simulink library "MCHP_Blockset"  (Simulink 7.5)
settings: Solver=ode45  SolverMode=SingleTasking  StartTime=0.0  StopTime=10.0  RelTol=1e-3
InitFcn:
  | disp('MCHP_Blockset_Library_InitFunction');
undefined symbols (not defined in the file): A0, A2, AD0, AVdd, B1, B5, B9, C10, C2, CMP2A, CMP3A, CMP4A, EXTREF1, EXTREF2, gcbh, MaxPer, MCHP_ACC_SAMx_Callback, MCHP_ADC_Callback, MCHP_ADC_HighSpeed_SAR_Callback, MCHP_ADC_HighSpeed_SAR_dsPIC_Callback, MCHP_ADC_SAME5x_Callback, MCHP_AFEC_SAM7x_Callback, MCHP_BUS_I2C_MASTER_callback, MCHP_BUS_SPI_callback, MCHP_C_function_Call_callback, MCHP_CN_Callback, MCHP_COMPARATOR1_callback, MCHP_CompilerOptimisation_Callback, MCHP_DACC_SAMx_Callback, MCHP_Digital_Input_Callback, MCHP_Digital_Output_Read_Callback, MCHP_Digital_Output_Write_Callback, MCHP_Fun, MCHP_HighSpeed_AnalogComparator_Callback, MCHP_IC_Callback, MCHP_IdleTask_Callback, MCHP_Interrupt_Callback, MCHP_Master_Callback, MCHP_MCPWM_Callback, MCHP_MCU_LOAD_Callback, MCHP_MCU_OVERLOAD_Callback, MCHP_MSI_Callback, MCHP_OC_HW_Callback, MCHP_OC_SW_Callback, MCHP_OP_AMP_Callback, MCHP_OrderInOut, MCHP_PDEC_Callback, MCHP_PGA_Callback, MCHP_PWM_Callback, MCHP_PWM_HighSpeed_Override_Callback, MCHP_PWM_HS_FEP_Callback, MCHP_PWM_SAM7x_Callback, MCHP_PWM_SAM7x_Override_Callback, MCHP_QDEC_SAMx_Callback, MCHP_QEI_Callback, MCHP_Scheduler_Options_Callback, MCHP_SECONDARY_CORE_Callback, MCHP_Tasks_State_Callback, MCHP_TCC_PWM_Callback, MCHP_TIMER_Config_Callback ... (+18)
libraries: MCHP_Blockset x2
(part 6 of 9)

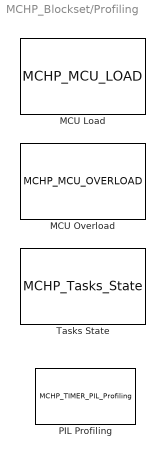
== system MCHP_Blockset/Profiling ==
  MCU Load : S-Function  InitFcn=MCHP_MCU_LOAD_Callback(gcbh,'InitFcn');  FunctionName=MCHP_MCU_LOAD  Parameters=[],MCHP_MCU_LOAD_Callback(gcbh,'S_OUTPUT'),[],MCHP_MCU_LOAD_Callback(gcbh,'S_OUTPUT_Size'),[],MCHP_MCU_LOAD_Callback(gcbh,'S_SampleTime'),0  EnableBusSupport=off  mask(MCU Load (Profile execution time)){MCULoadPin=Dynamic Options, MCULoadPin_TXT=A0 / Pin[17], MCULoadMeasure=on, TIMER_Resolution=Dynamic Options, TIMER_Resolution_TXT=Resol: 0.1143(us)  -  Max: 7.49(ms), MCHP_PORT={MCU Load Pin}{MCU_Load}0:1:A0;, MCHP_TIMER_REQUEST={MCU_Load}{MCU_Load}21:5:0:0:[]:524288;, MCHP_TIMER_RESULT=[2 65535 ], MCHP_MASTERLINK=UTester_33EP512MU810_CPULoad/Microchip Master, MCHP_COMPILED_INFO=CompiledSampleTime= [0.001   0 ];CompiledInportDataTypes=[ ];CompiledInportDataWidth=[];, Info=Timer 2:  Resol: 114.2857143(ns)  -  Max: 7.48983(ms), SampleTime=-1}
      mask prompts: MCULoadPin "MCU Load output PIN"; MCULoadMeasure "Output mcu load measurement"; TIMER_Resolution "Measure resolution"; Info "Timer info:"; SampleTime "Sample Time"
      mask help:
      | An output Pin is set high when CPU is busy: running time step calculation or a handling mcu interrupts.
      |
      | Busy time can be precisely quantified:
      | - in multitasking mode, the measurement trigger is the beginning of the task (sampling time) this block belong to.
      |
      | - in singletasking mode, the measurement trigger is the beginning of the groupe tasks which are triggered with this block.
      mask init:
      | MCHP_MCU_LOAD_Callback(gcbh,'INITIALISATION');
      settings: CopyFcn=MCHP_MCU_LOAD_Callback(gcbh,'CopyFcn');  PreSaveFcn=MCHP_Fun.PreSaveFcn_DynamicOptions(gcbh);  OpenFcn=MCHP_MCU_LOAD_Callback(gcbh,'OPEN');
      mask StyleString: popup(Dynamic Options),edit,checkbox,popup(Dynamic Options),edit,edit,edit,edit,edit,edit,edit,edit
      mask CallbackString: %MCHP_MCU_LOAD_Callback(gcbh,'MCULoadPin');||MCHP_MCU_LOAD_Callback(gcbh,'MCULoadMeasure');|MCHP_Fun.BlockUpdate(gcbh);||||||||
      mask Display:
      | MCHP_DrawLogo;disp('MCU Load\nLsb= 114.3(ns)\nA0');
      | port_label('output', 1 ,'L');
  MCU Overload : S-Function  InitFcn=MCHP_MCU_OVERLOAD_Callback(gcbh,'InitFcn');  FunctionName=MCHP_MCU_OVERLOAD  Parameters=[],MCHP_MCU_OVERLOAD_Callback(gcbh,'S_OUTPUT'),[],MCHP_MCU_OVERLOAD_Callback(gcbh,'S_OUTPUT_Size'),[],MCHP_MCU_OVERLOAD_Callback(gcbh,'S_SampleTime'),0  EnableBusSupport=off  mask(MCU Over-Load (Profile execution time)){MCUOverloadBlockOutput=on, MCUOverLoadPin=Dynamic Options, MCUOverLoadPin_TXT=None, MCHP_PORT=, MCHP_MASTERLINK=UTester_33EP512MU810_CPUOverLoad/Microchip Master, SampleTime=.001}
      mask prompts: MCUOverloadBlockOutput "Enable Block Output"; MCUOverLoadPin "MCU Overload PIN (asynchronously set to 1)"; SampleTime "Sample Time"
      mask help:
      | Block output is 0 when no overload has occured. Overload status is reset when block output is read.
      |
      | When an overload occurs, block output bit index represent overload for TID index.
      | bit 0 represent TID 0 (Fastest rate)
      | bit 1 represent TID 1 if it exist etc...
      | bit 15 represent TID 15 and higher
      |
      | Output pin is set to 1 asynchronously when an overload occurs. It remains equal to 1 and might be reset to 0 (Synchronously) using a digital Output block.
      mask init:
      | MCHP_MCU_OVERLOAD_Callback(gcbh,'INITIALISATION');
      settings: CopyFcn=MCHP_MCU_OVERLOAD_Callback(gcbh,'CopyFcn');  PreSaveFcn=MCHP_Fun.PreSaveFcn_DynamicOptions(gcbh);  OpenFcn=MCHP_MCU_OVERLOAD_Callback(gcbh,'OPEN');
      mask StyleString: checkbox,popup(Dynamic Options),edit,edit,edit,edit
      mask CallbackString: %MCHP_MCU_OVERLOAD_Callback(gcbh,'MCUOverloadBlockOutput');|%MCHP_MCU_OVERLOAD_Callback(gcbh,'MCUOverLoadPin');||||
      mask Display:
      | MCHP_DrawLogo;disp('MCU Over-Load');
      | port_label('output', 1 ,' ');
  PIL Profiling : S-Function  InitFcn=MCHP_TIMER_PIL_Profiling_Callback(gcbh,'InitFcn');  FunctionName=MCHP_TIMER_PIL_Profiling  EnableBusSupport=off  mask(Timer Configuration){TIMER_Ressource=Dynamic Options, TIMER_Ressource_TXT=No constraints [Prefered], TIMER_Ressource_Custom=[1], TIMER_Resolution=Dynamic Options, TIMER_Resolution_TXT=Resol: 32(us)  -  MaxPer: 2.1(s), MCHP_TIMER_REQUEST={TimerA}{TmrCfg}20:1:1:0:[]:4194304;, MCHP_TIMER_RESULT=[2 65535 ], MCHP_MASTERLINK=Timer_Config_30f4011/Microchip Master, Info=Timer 2}
      mask prompts: TIMER_Ressource "Timer Ressources"; TIMER_Ressource_TXT "Timer Ressources"; TIMER_Ressource_Custom "Timer List, example: [ 1  2  3  4  5 ]"; TIMER_Resolution "Resolution and max period"; Info "Timer info:"
      mask help:
      | Set Timer configuration
      | Peripheral that requrie a timer do not need this block. A timer is automatically assigned and configured in such case.
      mask init:
      | MCHP_TIMER_PIL_Profiling_Callback(gcbh,'INITIALISATION');
      settings: CopyFcn=MCHP_TIMER_PIL_Profiling_Callback(gcbh,'CopyFcn');  PreSaveFcn=MCHP_Fun.PreSaveFcn_DynamicOptions(gcbh);  OpenFcn=MCHP_TIMER_PIL_Profiling_Callback(gcbh,'OPEN');
      mask StyleString: popup(Dynamic Options),edit,edit,popup(Dynamic Options),edit,edit,edit,edit,edit
      mask CallbackString: MCHP_TIMER_PIL_Profiling_Callback(gcbh,'TIMER_Ressource');|||MCHP_TIMER_PIL_Profiling_Callback(gcbh,'TIMER_Resolution');|||||
      mask Display: MCHP_DrawLogo;disp('TIMER for PIL\nProfiling')
  Tasks State : S-Function  InitFcn=MCHP_Tasks_State_Callback(gcbh,'InitFcn');  FunctionName=MCHP_Tasks_State  Parameters=[],[],[],[],[],-1,0  EnableBusSupport=off  mask(MCU Over-Load (Profile execution time)){TasksPin=A[1:15], MCHP_PORT={Task D1 Running}{Task D1}15:1:A1;{Task D2 Running}{Task D2}15:1:A2;{Task D3 Running}{Task D3}15:1:A3;{Task D4 Running}{Task D4}15:1:A4;{Task D5 Running}{Task D5}15:1:A5;{Task D6 Running}{Task D6}15:1:A6;{Task D7 Running}{Task D7}15:1:A7;{Task D8 Running}{Task D8}15:1:A9;{Task D9 Running}{Task D9}15:1:A10;{Task D10 Running}{Task D10}15:1:A14;{Task D11 Running}{Task D11}15:1:A15;, MCHP_MASTERLINK=UTester_33EP512MU810_CPUOverLoad/Microchip Master}
      mask prompts: TasksPin "Running tasks pin list output ; example: A0 A1 A[5:8] B2..."
      mask help:
      | For each tasks, the corresponding pin is high when
      |  - the task is running or
      |  - the task execution is not finished but interrupted by an higher priority task
      | and set low otherwise
      |    First pin of the list is the state for the higher rate/priority task. (hit ctrl-j from model to show tasks list)
      | Value -1 will not affect a pin for the corresponding task.
      |
      | Task List updated with last model build
      | D1 => 1 (ms) ->  pin A1
      | D2 => 2 (ms) ->  pin A2
      | D3 => 4 (ms) ->  pin A3
      | D4 => 4  {+1} (ms) ->  pin A4
      | D5 => 20 (ms) ->  pin A5
      |
      | Available pins:
      |          A  [0   1   2   3   4   5   6   7   9  10  14  15]
      |          B  [0 : 15]
      |          C  [1   2   3   4  12  13  14  15]
      |          D  [0 : 15]
      |          E  [0 : 9]
      |          F  [0   1   2   3   4   5   8  12  13]
      |          G  [0   1   2   3   6   7   8   9  12  13  14  15]
      mask init:
      | MCHP_Tasks_State_Callback(gcbh,'INITIALISATION');
      settings: CopyFcn=MCHP_Tasks_State_Callback(gcbh,'CopyFcn');  OpenFcn=MCHP_Tasks_State_Callback(gcbh,'OPEN');
      mask Display: MCHP_DrawLogo;disp('Tasks State');

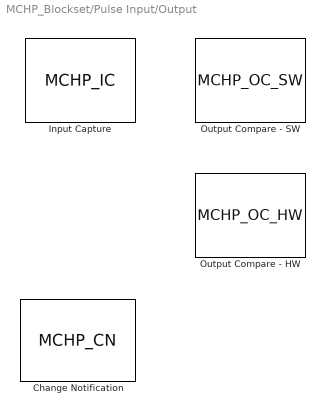
== system MCHP_Blockset/Pulse Input/Output ==
  Change Notification : S-Function  LoadFcn=MCHP_Fun.Load_EvalIn_ws(gcbh);  FunctionName=MCHP_CN  Parameters=SampleTime,MCHP_CN_Callback(gcbh,'S_INPUT'),MCHP_CN_Callback(gcbh,'S_OUTPUT'),0  EnableBusSupport=off  mask(Input driver for Change Notification Peripheral){IntPriority=6, Channel=[0     1     2], Channel_EP=[  C14  C13  B0 ], Channel_OLD=[0     1     2], Channel_UP_Down_Periode=[1     1     1], MaxChannel=[0.001   0.001   0.001], SafeMarge=[10    10    10], MaxChannelValue=2.^[ 13.966  13.966  13.966]  =>  [15999  15999  15999], CNxmax=[15999  15999  15999], Timer=[1  1  1], ChangeDetected=[0     0     0], OutputPortValue=[0     0     0], evalin_ws='', SampleTime=-1, Status=OK, MCHP_PORT={Change Notification 0}{CN0}9:0:C14;{Change Notification 1}{CN1}9:0:C13;{Change Notification 2}{CN2}9:0:B0;, MCHP_TIMER_REQUEST={Change Notification 0}{CN0}7:1:1:0:[]:17600;{Change Notification 1}{CN1}7:1:1:0:[]:17600;{Change Notification 2}{CN2}7:1:1:0:[]:17600;, MCHP_TIMER_RESULT=[2 17598.999999999996 ;2 17598.999999999996 ;2 17598.999999999996 ], MCHP_USER_INTERRUPTS={CNIE}{CN}{Change Notification}{6}, MCHP_MASTERLINK=Dvpt_CN/Microchip Master}
      mask prompts: IntPriority "Interrupt Priority  ( 1:lowest  7:Highest )"; Channel "CN Channels : [ 0  1  2  3  4  5  6  7 ]"; Channel_EP "CN Port : [  A0  A1  A2   ...   C7  C8  C9  ]"; Channel_OLD "internal"; Channel_UP_Down_Periode "Channel measurement type ; see above, within {1 2 3 4 5 8 10}"; MaxChannel "Max measured time / Channels"; SafeMarge "Safety margin in % (secure from overflow)"; MaxChannelValue "{'CN0max'  'CN1max'  'CN2max' } variables represent max time above ->"; CNxmax "CNxmax raw value"; ChangeDetected "Change Detected on   (0:None,  1:Rising edge, 2:Falling edge,  3:Both)"; OutputPortValue "Output Port Value"
      mask help:
      | Change Notification measure time :
      | 0 : no Measurements (for change detect only)
      | 1 : up
      | 2 : down
      | 3 : up & down
      | 4 : periode on rising edge
      | 8 : periode on falling edge
      | 5 : up & periode on rising edge
      | 10 : down & periode on falling edge
      |
      | CN Channels: [ 0  1  2  3  4  5  6  7 ]
      | CN Ports:      [  C14 C13 B0 B1 B2 B3 B4 B5 ]
      | CN Pins:       [ 16  15   2   3   4   5   6   7 ]
      mask init:
      | MCHP_CN_Callback(gcbh,'INITIALISATION');
      settings: PreSaveFcn=MCHP_Fun.PreSaveFcn_DynamicOptions(gcbh);  OpenFcn=MCHP_CN_Callback(gcbh,'OPEN');
      mask StyleString: popup(1|2|3|4|5|6|7),edit,edit,edit,edit,edit,edit,edit,edit,edit,edit,edit,edit,edit,edit,edit,edit,edit,edit,edit
      mask CallbackString: |MCHP_Fun.BlockUpdate(gcbh);|MCHP_Fun.BlockUpdate(gcbh);||MCHP_Fun.BlockUpdate(gcbh);||||||MCHP_Fun.BlockUpdate(gcbh);|MCHP_Fun.BlockUpdate(gcbh);||||||||
      mask Display:
      | MCHP_DrawLogo;color('blue');fprintf('CN        ');color('black');
      | 
      | port_label('output',1,'CN0_Up');
      | port_label('output',2,'CN1_Up');
      | port_label('output',3,'CN2_Up');
  Input Capture : S-Function  LoadFcn=MCHP_Fun.Load_EvalIn_ws(gcbh);  FunctionName=MCHP_IC  Parameters=SampleTime,MCHP_IC_Callback(gcbh,'S_INPUT'),MCHP_IC_Callback(gcbh,'S_OUTPUT'),0  EnableBusSupport=off  mask(Input driver for Input Capture Peripheral){IntPriority=4, Channel=[1     2], Channel_OLD=[1     2], PIN_IC1=Dynamic Options, PIN_IC1_TXT=Dynamic Options, PIN_IC2=Dynamic Options, PIN_IC2_TXT=Dynamic Options, PIN_IC3=Dynamic Options, PIN_IC3_TXT=Dynamic Options, PIN_IC4=Dynamic Options, PIN_IC4_TXT=Dynamic Options, PIN_IC5=Dynamic Options, PIN_IC5_TXT=Dynamic Options, PIN_IC6=Dynamic Options, PIN_IC6_TXT=Dynamic Options, PIN_IC7=Dynamic Options, PIN_IC7_TXT=Dynamic Options, PIN_IC8=Dynamic Options, PIN_IC8_TXT=Dynamic Options, PIN_IC9=Dynamic Options, PIN_IC9_TXT=Dynamic Options, PIN_IC10=Dynamic Options, PIN_IC10_TXT=Dynamic Options, PIN_IC11=Dynamic Options, PIN_IC11_TXT=Dynamic Options, PIN_IC12=Dynamic Options, PIN_IC12_TXT=Dynamic Options, PIN_IC13=Dynamic Options, PIN_IC13_TXT=Dynamic Options, PIN_IC14=Dynamic Options, PIN_IC14_TXT=Dynamic Options, PIN_IC15=Dynamic Options, PIN_IC15_TXT=Dynamic Options, PIN_IC16=Dynamic Options, PIN_IC16_TXT=Dynamic Options, Channel_UP_Down_Periode=[1     5], MaxChannel=[0.001     0.1], SafeMarge=[0     0], MaxChannelValue=2.^[ 7.960  14.610]  =>  [249  24999], ICxmax=[249  24999], Timer=[2  2], ChangeDetected=[0     0], ChangeDetectedPortRef=3, SampleTime=-1, evalin_ws='', Status=OK, MCHP_PORT={Input Capture 1}{IC1}6:0:D0;{Input Capture 2}{IC2}6:0:D1;, MCHP_TIMER_REQUEST={Input Capture 1}{IC1}6:1:1:0:[2  3]:16000;{Input Capture 2}{IC2}6:1:1:0:[2  3]:1600000;, MCHP_TIMER_RESULT=[2 15999 ;3 24999.000000000007 ], MCHP_MASTERLINK=Dvpt_IC/Microchip Master}
      mask prompts: IntPriority "Interrupt Priority  ( 1:lowest  7:Highest )"; Channel "Input Capture Channels : [ 1  2  7  8 ]"; Channel_OLD "internal"; PIN_IC1 "PIN for Input Capture 1 :"; PIN_IC1_TXT "internal"; PIN_IC2 "PIN for Input Capture 2 :"; PIN_IC2_TXT "internal"; PIN_IC3 "PIN for Input Capture 3 :"; PIN_IC3_TXT "internal"; PIN_IC4 "PIN for Input Capture 4 :"; PIN_IC4_TXT "internal"; PIN_IC5 "PIN for Input Capture 5 :"; PIN_IC5_TXT "internal"; PIN_IC6 "PIN for Input Capture 6 :"; PIN_IC6_TXT "internal"; PIN_IC7 "PIN for Input Capture 7 :"; PIN_IC7_TXT "internal"; PIN_IC8 "PIN for Input Capture 8 :"; PIN_IC8_TXT "internal"; PIN_IC9 "PIN for Input Capture 9 :"; PIN_IC9_TXT "internal"; PIN_IC10 "PIN for Input Capture 10 :"; PIN_IC10_TXT "internal"; PIN_IC11 "PIN for Input Capture 11 :"; PIN_IC11_TXT "internal"; PIN_IC12 "PIN for Input Capture 12 :"; PIN_IC12_TXT "internal"; PIN_IC13 "PIN for Input Capture 13 :"; PIN_IC13_TXT "internal"; PIN_IC14 "PIN for Input Capture 14 :"; PIN_IC14_TXT "internal"; PIN_IC15 "PIN for Input Capture 15 :"; PIN_IC15_TXT "internal"; PIN_IC16 "PIN for Input Capture 16 :"; PIN_IC16_TXT "internal"; Channel_UP_Down_Periode "Channel measurement type ; see above, within {1 2 3 4 5 8 10}"; MaxChannel "Max measured time / Channels"; SafeMarge "Safety margin in % (secure from overflow)"; MaxChannelValue "{'IC1max'  'IC2max' } variables represent max time above ->"; ICxmax "ICxmax raw value"; ChangeDetected "Change Detected on   (0:None,  1:Rising edge, 2:Falling edge,  3:Both)"
      mask help:
      | Input Capture measure time :
      | 0 : no Measurements (for change detect only)
      | 1 : up
      | 2 : down
      | 3 : up & down
      | 4 : periode on rising edge
      | 8 : periode on falling edge
      | 5 : up & periode on rising edge
      | 10 : down & periode on falling edge
      |
      | Input Capture Channels: [ 1  2  7  8 ]
      | Input Capture Ports:      [  D0 D1 B4 B5 ]
      | Input Capture Pins:       [ 23  18   6   7 ]
      mask init:
      | MCHP_IC_Callback(gcbh,'INITIALISATION');
      settings: PreSaveFcn=MCHP_Fun.PreSaveFcn_DynamicOptions(gcbh);  OpenFcn=MCHP_IC_Callback(gcbh,'OPEN');
      mask StyleString: popup(1|2|3|4|5|6|7),edit,edit,popup(Dynamic Options),edit,popup(Dynamic Options),edit,popup(Dynamic Options),edit,popup(Dynamic Options),edit,popup(Dynamic Options),edit,popup(Dynamic Options),edit,popup(Dynamic Options),edit,popup(Dynamic Options),edit,popup(Dynamic Options),edit,popup(Dynamic Options),edit,popup(Dynamic Options),edit,popup(Dynamic Options),edit,popup(Dynamic Options),edit,popup(Dynamic Options),edit,popup(Dynamic Options),edit,popup(Dynamic Options),edit,edit,edit,edit,edit,edit,edit,edit,edit,edit,edit,edit,edit,edit,edit,edit
      mask CallbackString:
      | |MCHP_Fun.BlockUpdate(gcbh);||if ~strcmp(get_param(gcbh,'PIN_IC1'),get_param(gcbh,'PIN_IC1_TXT'))
      | MCHP_Fun.BlockUpdate(gcbh);;
      | end||if ~strcmp(get_param(gcbh,'PIN_IC2'),get_param(gcbh,'PIN_IC2_TXT'))
      | MCHP_Fun.BlockUpdate(gcbh);;
      | end||if ~strcmp(get_param(gcbh,'PIN_IC3'),get_param(gcbh,'PIN_IC3_TXT'))
      | MCHP_Fun.BlockUpdate(gcbh);;
      | end||if ~strcmp(get_param(gcbh,'PIN_IC4'),get_param(gcbh,'PIN_IC4_TXT'))
      | MCHP_Fun.BlockUpdate(gcbh);;
      | end||if ~strcmp(get_param(gcbh,'PIN_IC5'),get_param(gcbh,'PIN_IC5_TXT'))
      | MCHP_Fun.BlockUpdate(gcbh);;
      | end||if ~strcmp(get_param(gcbh,'PIN_IC6'),get_param(gcbh,'PIN_IC6_TXT'))
      | MCHP_Fun.BlockUpdate(gcbh);;
      | end||if ~strcmp(get_param(gcbh,'PIN_IC7'),get_param(gcbh,'PIN_IC7_TXT'))
      | MCHP_Fun.BlockUpdate(gcbh);;
      | end||if ~strcmp(get_param(gcbh,'PIN_IC8'),get_param(gcbh,'PIN_IC8_TXT'))
      | MCHP_Fun.BlockUpdate(gcbh);;
      | end||if ~strcmp(get_param(gcbh,'PIN_IC9'),get_param(gcbh,'PIN_IC9_TXT'))
      | MCHP_Fun.BlockUpdate(gcbh);;
      | end||if ~strcmp(get_param(gcbh,'PIN_IC10'),get_param(gcbh,'PIN_IC10_TXT'))
      | MCHP_Fun.BlockUpdate(gcbh);;
      | end||if ~strcmp(get_param(gcbh,'PIN_IC11'),get_param(gcbh,'PIN_IC11_TXT'))
      | MCHP_Fun.BlockUpdate(gcbh);;
      | end||if ~strcmp(get_param(gcbh,'PIN_IC12'),get_param(gcbh,'PIN_IC12_TXT'))
      | MCHP_Fun.BlockUpdate(gcbh);;
      | end||if ~strcmp(get_param(gcbh,'PIN_IC13'),get_param(gcbh,'PIN_IC13_TXT'))
      | MCHP_Fun.BlockUpdate(gcbh);;
      | end||if ~strcmp(get_param(gcbh,'PIN_IC14'),get_param(gcbh,'PIN_IC14_TXT'))
      | MCHP_Fun.BlockUpdate(gcbh);;
      | end||if ~strcmp(get_param(gcbh,'PIN_IC15'),get_param(gcbh,'PIN_IC15_TXT'))
      | MCHP_Fun.BlockUpdate(gcbh);;
      | end||if ~strcmp(get_param(gcbh,'PIN_IC16'),get_param(gcbh,'PIN_IC16_TXT'))
      | MCHP_Fun.BlockUpdate(gcbh);;
      | end||MCHP_Fun.BlockUpdate(gcbh);||||||MCHP_Fun.BlockUpdate(gcbh);||||||||
      mask Display:
      | MCHP_DrawLogo;color('blue');fprintf('IC        ');color('black');
      | 
      | port_label('output',1,'IC1_Up');
      | port_label('output',2,'IC2_Up');
      | port_label('output',3,'IC2_Per');
  Output Compare - HW : S-Function  LoadFcn=MCHP_Fun.Load_EvalIn_ws(gcbh);  FunctionName=MCHP_OC_HW  Parameters=SampleTime,MCHP_OC_HW_Callback(gcbh,'S_INPUT'),MCHP_OC_HW_Callback(gcbh,'S_OUTPUT'),0  EnableBusSupport=off  mask(Input driver for Output Compare Peripheral Hardware){Channel=[1     2     3], Channel_OLD=[1     2     3], PIN_OC1_TXT=Dynamic Options, PIN_OC2_TXT=Dynamic Options, PIN_OC3_TXT=Dynamic Options, PIN_OC4_TXT=Dynamic Options, PIN_OC5_TXT=Dynamic Options, PIN_OC6_TXT=Dynamic Options, PIN_OC7_TXT=Dynamic Options, PIN_OC8_TXT=Dynamic Options, PIN_OC9_TXT=Dynamic Options, PIN_OC10_TXT=Dynamic Options, PIN_OC11_TXT=Dynamic Options, PIN_OC12_TXT=Dynamic Options, PIN_OC13_TXT=Dynamic Options, PIN_OC14_TXT=Dynamic Options, PIN_OC15_TXT=Dynamic Options, PIN_OC16_TXT=Dynamic Options, PIN_OCFA_TXT=Dynamic Options, PIN_OCFB_TXT=Dynamic Options, PIN_OCFC_TXT=Dynamic Options, Channel_UP_Down_Periode=[5    10     5], PulseTrig=Continuous pulses, InputPeriod=are set to the Max time (constant below), MaxChannel=[0.0001   0.0001   0.0001], MaxChannelUnique=.0001, MaxChannelValue=2.^[ 10.965  10.965  10.965]  =>  [1999  1999  1999], OCxmax=[1999  1999  1999], Timer=[-2 -2 -2], evalin_ws='', SampleTime=-1, MCHP_PORT={Output Compare 1}{OC1}7:1:P55;{Output Compare 2}{OC2}7:1:P56;{Output Compare 3}{OC3}7:1:P57;, MCHP_TIMER_REQUEST=, MCHP_TIMER_RESULT=[ ], MCHP_MASTERLINK=Dvpt_OC_HW/Microchip Master, PIN_OC1=Dynamic Options, PIN_OC2=Dynamic Options, PIN_OC3=Dynamic Options, PIN_OC4=Dynamic Options, PIN_OC5=Dynamic Options, PIN_OC6=Dynamic Options, PIN_OC7=Dynamic Options, PIN_OC8=Dynamic Options, PIN_OC9=Dynamic Options, PIN_OC10=Dynamic Options, PIN_OC11=Dynamic Options, PIN_OC12=Dynamic Options, PIN_OC13=Dynamic Options, PIN_OC14=Dynamic Options, PIN_OC15=Dynamic Options, PIN_OC16=Dynamic Options, PIN_OCFA=Dynamic Options, PIN_OCFB=Dynamic Options, PIN_OCFC=Dynamic Options}
      mask prompts: Channel "Output Compare Channels : [ 1  2  3  4 ]"; Channel_OLD "internal"; PIN_OC1_TXT "internal"; PIN_OC2_TXT "internal"; PIN_OC3_TXT "internal"; PIN_OC4_TXT "internal"; PIN_OC5_TXT "internal"; PIN_OC6_TXT "internal"; PIN_OC7_TXT "internal"; PIN_OC8_TXT "internal"; PIN_OC9_TXT "internal"; PIN_OC10_TXT "internal"; PIN_OC11_TXT "internal"; PIN_OC12_TXT "internal"; PIN_OC13_TXT "internal"; PIN_OC14_TXT "internal"; PIN_OC15_TXT "internal"; PIN_OC16_TXT "internal"; PIN_OCFA_TXT "internal"; PIN_OCFB_TXT "internal"; PIN_OCFC_TXT "internal"; Channel_UP_Down_Periode "Channel measurement type ; see above, within {5}"; PulseTrig "Mode"; InputPeriod "Period"; MaxChannel "Max time / Channels"; MaxChannelUnique "Max Time for all channels"; MaxChannelValue "{'OC1max'  'OC2max'  'OC3max' } variables represent max time above ->"; OCxmax "OCxmax raw value"; PIN_OC1 "PIN for Output Compare 1 :"; PIN_OC2 "PIN for Output Compare 2 :"; PIN_OC3 "PIN for Output Compare 3 :"; PIN_OC4 "PIN for Output Compare 4 :"; PIN_OC5 "PIN for Output Compare 5 :"; PIN_OC6 "PIN for Output Compare 6 :"; PIN_OC7 "PIN for Output Compare 7 :"; PIN_OC8 "PIN for Output Compare 8 :"; PIN_OC9 "PIN for Output Compare 9 :"; PIN_OC10 "PIN for Output Compare 10 :"; PIN_OC11 "PIN for Output Compare 11 :"; PIN_OC12 "PIN for Output Compare 12 :"; PIN_OC13 "PIN for Output Compare 13 :"; PIN_OC14 "PIN for Output Compare 14 :"; PIN_OC15 "PIN for Output Compare 15 :"; PIN_OC16 "PIN for Output Compare 16 :"; PIN_OCFA "PIN for Output Compare Fault A:"; PIN_OCFB "PIN for Output Compare Fault B:"; PIN_OCFC "PIN for Output Compare Fault C:"
      mask help:
      | Output Compare Setting :
      | 5 : up & periode
      | 10 : down & periode
      |
      |
      | Output Compare Channels: [ 1 2 3 4 ]
      | Output Compare Pins are remapables.
      mask init:
      | MCHP_OC_HW_Callback(gcbh,'INITIALISATION');
      settings: PreSaveFcn=MCHP_Fun.PreSaveFcn_DynamicOptions(gcbh);  OpenFcn=MCHP_OC_HW_Callback(gcbh,'OPEN');
      mask StyleString: edit,edit,edit,edit,edit,edit,edit,edit,edit,edit,edit,edit,edit,edit,edit,edit,edit,edit,edit,edit,edit,edit,popup(Continuous pulses|Single pulse triggered by block execution|Single pulse triggered by independant block input),popup(are set to the Max time (constant below)|are independants block inputs|are one unique block input),edit,edit,edit,edit,edit,edit,edit,edit,edit,edit,edit,popup(Dynamic Options),popup(Dynamic Options),popup(Dynamic Options),popup(Dynamic Options),popup(Dynamic Options),popup(Dynamic Options),popup(Dynamic Options),popup(Dynamic Options),popup(Dynamic Options),popup(Dynamic Options),popup(Dynamic Options),popup(Dynamic Options),popup(Dynamic Options),popup(Dynamic Options),popup(Dynamic Options),popup(Dynamic Options),popup(Dynamic Options),popup(Dynamic Options),popup(Dynamic Options)
      mask CallbackString:
      | MCHP_Fun.BlockUpdate(gcbh);|||||||||||||||||||||MCHP_Fun.BlockUpdate(gcbh);||||||||||||||if ~strcmp(get_param(gcbh,'PIN_OC1'),get_param(gcbh,'PIN_OC1_TXT'))
      | MCHP_Fun.BlockUpdate(gcbh);
      | end|if ~strcmp(get_param(gcbh,'PIN_OC2'),get_param(gcbh,'PIN_OC2_TXT'))
      | MCHP_Fun.BlockUpdate(gcbh);
      | end|if ~strcmp(get_param(gcbh,'PIN_OC3'),get_param(gcbh,'PIN_OC3_TXT'))
      | MCHP_Fun.BlockUpdate(gcbh);
      | end|if ~strcmp(get_param(gcbh,'PIN_OC4'),get_param(gcbh,'PIN_OC4_TXT'))
      | MCHP_Fun.BlockUpdate(gcbh);
      | end|if ~strcmp(get_param(gcbh,'PIN_OC5'),get_param(gcbh,'PIN_OC5_TXT'))
      | MCHP_Fun.BlockUpdate(gcbh);
      | end|if ~strcmp(get_param(gcbh,'PIN_OC6'),get_param(gcbh,'PIN_OC6_TXT'))
      | MCHP_Fun.BlockUpdate(gcbh);
      | end|if ~strcmp(get_param(gcbh,'PIN_OC7'),get_param(gcbh,'PIN_OC7_TXT'))
      | MCHP_Fun.BlockUpdate(gcbh);
      | end|if ~strcmp(get_param(gcbh,'PIN_OC8'),get_param(gcbh,'PIN_OC8_TXT'))
      | MCHP_Fun.BlockUpdate(gcbh);
      | end|if ~strcmp(get_param(gcbh,'PIN_OC9'),get_param(gcbh,'PIN_OC9_TXT'))
      | MCHP_Fun.BlockUpdate(gcbh);
      | end|if ~strcmp(get_param(gcbh,'PIN_OC10'),get_param(gcbh,'PIN_OC10_TXT'))
      | MCHP_Fun.BlockUpdate(gcbh);
      | end|if ~strcmp(get_param(gcbh,'PIN_OC11'),get_param(gcbh,'PIN_OC11_TXT'))
      | MCHP_Fun.BlockUpdate(gcbh);
      | end|if ~strcmp(get_param(gcbh,'PIN_OC12'),get_param(gcbh,'PIN_OC12_TXT'))
      | MCHP_Fun.BlockUpdate(gcbh);
      | end|if ~strcmp(get_param(gcbh,'PIN_OC13'),get_param(gcbh,'PIN_OC13_TXT'))
      | MCHP_Fun.BlockUpdate(gcbh);
      | end|if ~strcmp(get_param(gcbh,'PIN_OC14'),get_param(gcbh,'PIN_OC14_TXT'))
      | MCHP_Fun.BlockUpdate(gcbh);
      | end|if ~strcmp(get_param(gcbh,'PIN_OC15'),get_param(gcbh,'PIN_OC15_TXT'))
      | MCHP_Fun.BlockUpdate(gcbh);
      | end|if ~strcmp(get_param(gcbh,'PIN_OC16'),get_param(gcbh,'PIN_OC16_TXT'))
      | MCHP_Fun.BlockUpdate(gcbh);
      | end|if ~strcmp(get_param(gcbh,'PIN_OCFA'),get_param(gcbh,'PIN_OCFA_TXT'))
      | MCHP_Fun.BlockUpdate(gcbh);
      | end|if ~strcmp(get_param(gcbh,'PIN_OCFB'),get_param(gcbh,'PIN_OCFB_TXT'))
      | MCHP_Fun.BlockUpdate(gcbh);
      | end|if ~strcmp(get_param(gcbh,'PIN_OCFC'),get_param(gcbh,'PIN_OCFC_TXT'))
      | MCHP_Fun.BlockUpdate(gcbh);
      | end
      mask TabNameString: Main,Main,Main,Main,Main,Main,Main,Main,Main,Main,Main,Main,Main,Main,Main,Main,Main,Main,Main,Main,Main,Main,Main,Main,Main,Main,Main,Main,Main,Main,Main,Main,Main,Main,Main,Pin Maping,Pin Maping,Pin Maping,Pin Maping,Pin Maping,Pin Maping,Pin Maping,Pin Maping,Pin Maping,Pin Maping,Pin Maping,Pin Maping,Pin Maping,Pin Maping,Pin Maping,Pin Maping,Pin Maping,Pin Maping,Pin Maping
      mask Display:
      | MCHP_DrawLogo;color('blue');fprintf('        OC\n        (hw)');color('black');
      | 
      | port_label('input',1,'OC1_Up');
      | port_label('input',2,'OC2_Down');
      | port_label('input',3,'OC3_Up');
  Output Compare - SW : S-Function  LoadFcn=MCHP_Fun.Load_EvalIn_ws(gcbh);  FunctionName=MCHP_OC_SW  Parameters=SampleTime,MCHP_OC_SW_Callback(gcbh,'S_INPUT'),MCHP_OC_SW_Callback(gcbh,'S_OUTPUT'),0  EnableBusSupport=off  mask(Output driver for Output Compare Peripheral Software (Interrupt based)){IntPriority=3, Channel=[1     2     3], Channel_OLD=[1     2     3], PIN_OC1_TXT=Dynamic Options, PIN_OC2_TXT=Dynamic Options, PIN_OC3_TXT=Dynamic Options, PIN_OC4_TXT=Dynamic Options, PIN_OC5_TXT=Dynamic Options, PIN_OC6_TXT=Dynamic Options, PIN_OC7_TXT=Dynamic Options, PIN_OC8_TXT=Dynamic Options, PIN_OC9_TXT=Dynamic Options, PIN_OC10_TXT=Dynamic Options, PIN_OC11_TXT=Dynamic Options, PIN_OC12_TXT=Dynamic Options, PIN_OC13_TXT=Dynamic Options, PIN_OC14_TXT=Dynamic Options, PIN_OC15_TXT=Dynamic Options, PIN_OC16_TXT=Dynamic Options, Channel_UP_Down_Periode=[5     5    32], InputPeriod=is setup with the Max time, MaxChannel=[0.001   0.001    0.01], MaxChannelValue=2.^[ 14.288  14.288  14.610]  =>  [19999  19999  24999], OCxmax=[19999  19999  24999], Timer=[-2 -2  1], evalin_ws='', SampleTime=-1, Status=OK, MCHP_PORT={Output Compare 1}{OC1}7:1:P57;{Output Compare 2}{OC2}7:1:P56;{Output Compare 3}{OC3}7:1:P55;, MCHP_TIMER_REQUEST={Output Compare 1}{OC1}6:0:1:0:[1  2  3  4  5]:200000;, MCHP_TIMER_RESULT=[1 24999.000000000007 ], MCHP_MASTERLINK=Dvpt_OC_SW/Microchip Master, PIN_OC1=Dynamic Options, PIN_OC2=Dynamic Options, PIN_OC3=Dynamic Options, PIN_OC4=Dynamic Options, PIN_OC5=Dynamic Options, PIN_OC6=Dynamic Options, PIN_OC7=Dynamic Options, PIN_OC8=Dynamic Options, PIN_OC9=Dynamic Options, PIN_OC10=Dynamic Options, PIN_OC11=Dynamic Options, PIN_OC12=Dynamic Options, PIN_OC13=Dynamic Options, PIN_OC14=Dynamic Options, PIN_OC15=Dynamic Options, PIN_OC16=Dynamic Options}
      mask prompts: IntPriority "Interrupt Priority  ( 1:lowest  7:Highest )"; Channel "Output Compare Channels : [ 1  2  3  4 ]"; Channel_OLD "internal"; PIN_OC1_TXT "internal"; PIN_OC2_TXT "internal"; PIN_OC3_TXT "internal"; PIN_OC4_TXT "internal"; PIN_OC5_TXT "internal"; PIN_OC6_TXT "internal"; PIN_OC7_TXT "internal"; PIN_OC8_TXT "internal"; PIN_OC9_TXT "internal"; PIN_OC10_TXT "internal"; PIN_OC11_TXT "internal"; PIN_OC12_TXT "internal"; PIN_OC13_TXT "internal"; PIN_OC14_TXT "internal"; PIN_OC15_TXT "internal"; PIN_OC16_TXT "internal"; Channel_UP_Down_Periode "Channel measurement type ; see above, within { 3 5 10 32}"; InputPeriod "Period"; MaxChannel "Max time / Channels"; MaxChannelValue "{'OC1max'  'OC2max'  'OC3max' } variables represent max time above ->"; OCxmax "OCxmax raw value"; PIN_OC1 "PIN for Output Compare 1 :"; PIN_OC2 "PIN for Output Compare 2 :"; PIN_OC3 "PIN for Output Compare 3 :"; PIN_OC4 "PIN for Output Compare 4 :"; PIN_OC5 "PIN for Output Compare 5 :"; PIN_OC6 "PIN for Output Compare 6 :"; PIN_OC7 "PIN for Output Compare 7 :"; PIN_OC8 "PIN for Output Compare 8 :"; PIN_OC9 "PIN for Output Compare 9 :"; PIN_OC10 "PIN for Output Compare 10 :"; PIN_OC11 "PIN for Output Compare 11 :"; PIN_OC12 "PIN for Output Compare 12 :"; PIN_OC13 "PIN for Output Compare 13 :"; PIN_OC14 "PIN for Output Compare 14 :"; PIN_OC15 "PIN for Output Compare 15 :"; PIN_OC16 "PIN for Output Compare 16 :"
      mask help:
      | Output Compare Setting :
      | 3 : up & down
      | 5 : up & periode
      | 10 : down & periode
      | 32 : Toggle
      |
      | Minimum time is required between "events".
      | (avoid duty cycle near 0% and 100%. 0% and 100% Duty cycle are Ok.)
      |
      | Output Compare Channels: [ 1 2 3 4 ]
      | Output Compare Pins are remapables.
      mask init:
      | MCHP_OC_SW_Callback(gcbh,'INITIALISATION');
      settings: PreSaveFcn=MCHP_Fun.PreSaveFcn_DynamicOptions(gcbh);  OpenFcn=MCHP_OC_SW_Callback(gcbh,'OPEN');
      mask StyleString: popup(1|2|3|4|5|6|7),edit,edit,edit,edit,edit,edit,edit,edit,edit,edit,edit,edit,edit,edit,edit,edit,edit,edit,edit,popup(is a block input|is setup with the Max time),edit,edit,edit,edit,edit,edit,edit,edit,edit,edit,edit,popup(Dynamic Options),popup(Dynamic Options),popup(Dynamic Options),popup(Dynamic Options),popup(Dynamic Options),popup(Dynamic Options),popup(Dynamic Options),popup(Dynamic Options),popup(Dynamic Options),popup(Dynamic Options),popup(Dynamic Options),popup(Dynamic Options),popup(Dynamic Options),popup(Dynamic Options),popup(Dynamic Options),popup(Dynamic Options)
      mask CallbackString:
      | |MCHP_Fun.BlockUpdate(gcbh);||||||||||||||||||MCHP_Fun.BlockUpdate(gcbh);|||||||||||||if ~strcmp(get_param(gcbh,'PIN_OC1'),get_param(gcbh,'PIN_OC1_TXT'))
      | MCHP_Fun.BlockUpdate(gcbh);
      | end|if ~strcmp(get_param(gcbh,'PIN_OC2'),get_param(gcbh,'PIN_OC2_TXT'))
      | MCHP_Fun.BlockUpdate(gcbh);
      | end|if ~strcmp(get_param(gcbh,'PIN_OC3'),get_param(gcbh,'PIN_OC3_TXT'))
      | MCHP_Fun.BlockUpdate(gcbh);
      | end|if ~strcmp(get_param(gcbh,'PIN_OC4'),get_param(gcbh,'PIN_OC4_TXT'))
      | MCHP_Fun.BlockUpdate(gcbh);
      | end|if ~strcmp(get_param(gcbh,'PIN_OC5'),get_param(gcbh,'PIN_OC5_TXT'))
      | MCHP_Fun.BlockUpdate(gcbh);
      | end|if ~strcmp(get_param(gcbh,'PIN_OC6'),get_param(gcbh,'PIN_OC6_TXT'))
      | MCHP_Fun.BlockUpdate(gcbh);
      | end|if ~strcmp(get_param(gcbh,'PIN_OC7'),get_param(gcbh,'PIN_OC7_TXT'))
      | MCHP_Fun.BlockUpdate(gcbh);
      | end|if ~strcmp(get_param(gcbh,'PIN_OC8'),get_param(gcbh,'PIN_OC8_TXT'))
      | MCHP_Fun.BlockUpdate(gcbh);
      | end|if ~strcmp(get_param(gcbh,'PIN_OC9'),get_param(gcbh,'PIN_OC9_TXT'))
      | MCHP_Fun.BlockUpdate(gcbh);
      | end|if ~strcmp(get_param(gcbh,'PIN_OC10'),get_param(gcbh,'PIN_OC10_TXT'))
      | MCHP_Fun.BlockUpdate(gcbh);
      | end|if ~strcmp(get_param(gcbh,'PIN_OC11'),get_param(gcbh,'PIN_OC11_TXT'))
      | MCHP_Fun.BlockUpdate(gcbh);
      | end|if ~strcmp(get_param(gcbh,'PIN_OC12'),get_param(gcbh,'PIN_OC12_TXT'))
      | MCHP_Fun.BlockUpdate(gcbh);
      | end|if ~strcmp(get_param(gcbh,'PIN_OC13'),get_param(gcbh,'PIN_OC13_TXT'))
      | MCHP_Fun.BlockUpdate(gcbh);
      | end|if ~strcmp(get_param(gcbh,'PIN_OC14'),get_param(gcbh,'PIN_OC14_TXT'))
      | MCHP_Fun.BlockUpdate(gcbh);
      | end|if ~strcmp(get_param(gcbh,'PIN_OC15'),get_param(gcbh,'PIN_OC15_TXT'))
      | MCHP_Fun.BlockUpdate(gcbh);
      | end|if ~strcmp(get_param(gcbh,'PIN_OC16'),get_param(gcbh,'PIN_OC16_TXT'))
      | MCHP_Fun.BlockUpdate(gcbh);
      | end
      mask TabNameString: Main,Main,Main,Main,Main,Main,Main,Main,Main,Main,Main,Main,Main,Main,Main,Main,Main,Main,Main,Main,Main,Main,Main,Main,Main,Main,Main,Main,Main,Main,Main,Main,Pin Maping,Pin Maping,Pin Maping,Pin Maping,Pin Maping,Pin Maping,Pin Maping,Pin Maping,Pin Maping,Pin Maping,Pin Maping,Pin Maping,Pin Maping,Pin Maping,Pin Maping,Pin Maping
      mask Display:
      | MCHP_DrawLogo;color('blue');fprintf('        OC\n        (sw)');color('black');
      | 
      | port_label('input',1,'OC1_Up');
      | port_label('input',2,'OC2_Up');
      | port_label('input',3,'OC3_Toggle');
